simulink model "hex_out"  (Simulink 7.1)
settings: Solver=ode45  StartTime=0.0  StopTime=100000  RelTol=1e-3
InitFcn:
  | init
StartFcn:
  | init
libraries: xbsIndex_r4 x89
settings Model: Creator=sgupta  LastModifiedBy=sgupta

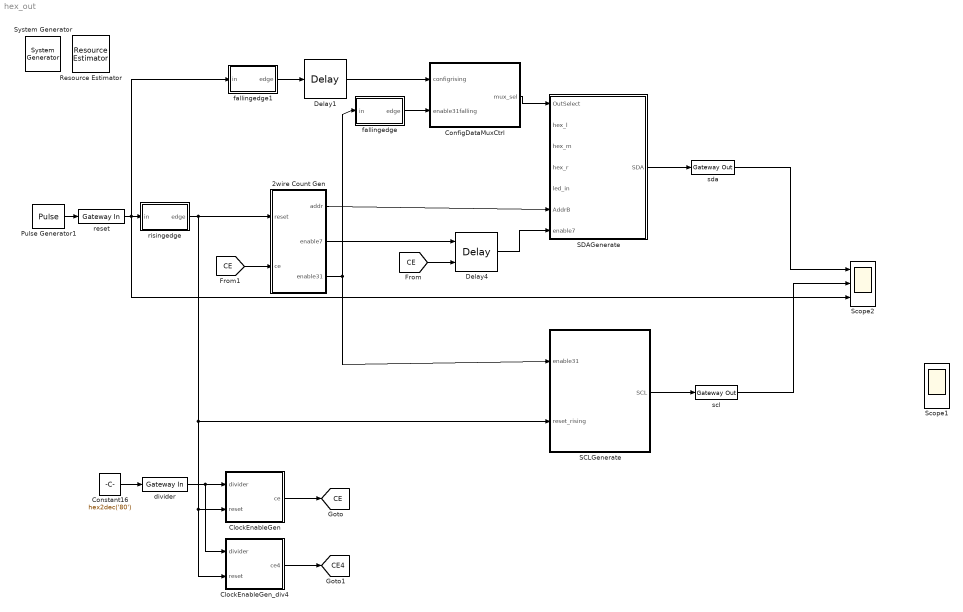
== system hex_out ==
  " System Generator" : xbsIndex_r4/ System Generator  Tag=genX  SystemSampleTime=-1  xilinxfamily=virtex4  part=xc4vfx100  speed=-11  package=ff1517  synthesis_tool=XST  clock_wrapper=Clock Enables  directory=./netlist02  testbench=off  simulink_period=1  sysclk_period=10  dcm_input_clock_period=100  incr_netlist=off  trim_vbits=Everywhere in SubSystem  dbl_ovrd=According to Block Masks  core_generation=According to Block Masks  run_coregen=off  deprecated_control=off  eval_field=0  block_type=sysgen
      settings: block_version=10.1.3
  2wire Count Gen : Subsystem
  ClockEnableGen : Subsystem
  ClockEnableGen_div4 : Subsystem
  ConfigDataMuxCtrl : Subsystem
  Constant16 : Constant  Value=hex2dec('80')  OutDataType=sfix(16)  OutScaling=2^0
  Delay1 : xbsIndex_r4/Delay  en=off  latency=80  dbl_ovrd=off  reg_retiming=off  block_type=delay
      settings: xl_area=[1 1 0 0 0 0 0]
  Delay4 : xbsIndex_r4/Delay  en=on  latency=1  dbl_ovrd=off  reg_retiming=off  block_type=delay
      settings: xl_area=[1 1 0 0 0 0 0]
  Pulse Generator1 : DiscretePulseGenerator  PulseType=Time based  Period=500000  PulseWidth=10/2000*100  PhaseDelay=2000
  Resource Estimator : xbsIndex_r4/Resource Estimator  Tag=resEstTag  Slices=127  FFs=89  BRAMs=0  LUTs=186  IOBs=57  EBMs=0  TBUFs=0  xl_use_estimator_area=off  est_options=Estimate  block_type=resource_estimator
      settings: AttributesFormatString=Resource\nEstimator  block_version=10.1.3
  SCLGenerate : Subsystem
  SDAGenerate : Subsystem
  Scope1 : Scope  NumInputPorts=3
      settings: TimeRange=30000  YMin=0~0~-1  YMax=1~1~1
  Scope2 : Scope  NumInputPorts=3
      settings: YMin=0~0~-1  YMax=1~1~1  SaveName=ScopeData2
  divider : xbsIndex_r4/Gateway In  arith_type=Unsigned  n_bits=8  bin_pt=0  quantization=Truncate  overflow=Wrap  period=1  dbl_ovrd=off  timing_constraint=None  locs_specified=off  LOCs={}  block_type=gatewayin
      settings: infoedit="Gateway in block.  Converts inputs of type Simulink integer, double and fixed point to  Xilinx fixed point type.<P><P>Hardware notes:  In hardware these blocks become top level input ports."  xl_area=[0 0 0 0 8 0 0]  block_version=10.1.3
  fallingedge : Subsystem
  fallingedge1 : Subsystem
  reset : xbsIndex_r4/Gateway In  arith_type=Boolean  n_bits=8  bin_pt=0  quantization=Truncate  overflow=Wrap  period=1  dbl_ovrd=off  timing_constraint=None  locs_specified=off  LOCs={}  block_type=gatewayin
      settings: infoedit="Gateway in block.  Converts inputs of type Simulink integer, double and fixed point to  Xilinx fixed point type.<P><P>Hardware notes:  In hardware these blocks become top level input ports."  xl_area=[0 0 0 0 1 0 0]  block_version=10.1.3
  risingedge : Subsystem
  scl : xbsIndex_r4/Gateway Out  hdl_port=on  timing_constraint=None  locs_specified=off  LOCs={}  block_type=gatewayout
      settings: infoedit="Gateway out block.  Converts Xilinx fixed point inputs into ouputs of type Simulink integer, double, or fixed point.<P><P>Hardware notes:  In hardware these blocks become top level output ports or are discarded, depending on how they are configured."  block_version=10.1.3
  sda : xbsIndex_r4/Gateway Out  hdl_port=on  timing_constraint=None  locs_specified=off  LOCs={}  block_type=gatewayout
      settings: infoedit="Gateway out block.  Converts Xilinx fixed point inputs into ouputs of type Simulink integer, double, or fixed point.<P><P>Hardware notes:  In hardware these blocks become top level output ports or are discarded, depending on how they are configured."  block_version=10.1.3
  tag scope: CE4=global, CE=global
  wires:
  2wire Count Gen/2(enable7) -> Delay4/1
  2wire Count Gen/3(enable31) -> fallingedge/1(in), SCLGenerate/1(enable31)
  divider/1 -> ClockEnableGen/1(divider), ClockEnableGen_div4/1(divider)
  Constant16/1 -> divider/1
  ClockEnableGen/1(ce) -> [CE]
  [CE] -> Delay4/2
  fallingedge/1(edge) -> ConfigDataMuxCtrl/2(enable31falling)
  ClockEnableGen_div4/1(ce4) -> [CE4]
  Delay4/1 -> SDAGenerate/7(enable7)
  2wire Count Gen/1(addr) -> SDAGenerate/6(AddrB)
  ConfigDataMuxCtrl/1(mux_sel) -> SDAGenerate/1(OutSelect)
  [CE] -> 2wire Count Gen/2(ce)
  SDAGenerate/1(SDA) -> sda/1
  SCLGenerate/1(SCL) -> scl/1
  sda/1 -> Scope2/1
  scl/1 -> Scope2/2
  Pulse Generator1/1 -> reset/1
  reset/1 -> Scope2/3, risingedge/1(in), fallingedge1/1(in)
  risingedge/1(edge) -> SCLGenerate/2(reset_rising), ClockEnableGen_div4/2(reset), ClockEnableGen/2(reset), 2wire Count Gen/1(reset)
  fallingedge1/1(edge) -> Delay1/1
  Delay1/1 -> ConfigDataMuxCtrl/1(configrising)

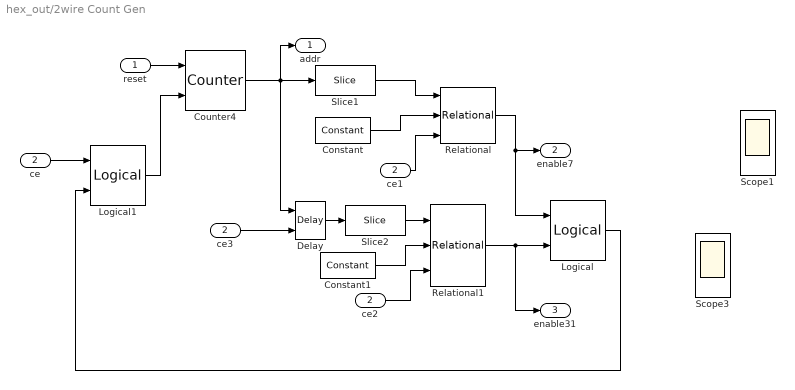
== system hex_out/2wire Count Gen ==
  reset : Inport
  ce : Inport  Port=2
  Constant : xbsIndex_r4/Constant  arith_type=Unsigned  const=7  n_bits=6  bin_pt=0  explicit_period=off  period=1  equ=P=C  opselect=C  inp2=PCIN>>17  opr=+  inp1=P  carry=CIN  dbl_ovrd=off  block_type=constant
  Constant1 : xbsIndex_r4/Constant  arith_type=Unsigned  const=31  n_bits=6  bin_pt=0  explicit_period=off  period=1  equ=P=C  opselect=C  inp2=PCIN>>17  opr=+  inp1=P  carry=CIN  dbl_ovrd=off  block_type=constant
  Counter4 : xbsIndex_r4/Counter  cnt_type=Free Running  cnt_to=23  operation=Up  start_count=0  cnt_by_val=1  arith_type=Unsigned  n_bits=6  bin_pt=0  load_pin=off  rst=on  en=on  explicit_period=on  period=1  dbl_ovrd=off  use_behavioral_HDL=off  use_rpm=off  implementation=Fabric  block_type=counter
      settings: xl_area=[4 6 0 6 0 0 0]
  Delay : xbsIndex_r4/Delay  en=on  latency=1  dbl_ovrd=off  reg_retiming=off  block_type=delay
      settings: xl_area=[3 6 0 0 0 0 0]
  Logical : xbsIndex_r4/Logical  logical_function=AND  inputs=2  en=off  latency=0  precision=Full  arith_type=Unsigned  n_bits=16  bin_pt=0  align_bp=on  dbl_ovrd=off  block_type=logical
      settings: xl_area=[1 0 0 1 0 0 0]
  Logical1 : xbsIndex_r4/Logical  logical_function=AND  inputs=2  en=off  latency=0  precision=Full  arith_type=Unsigned  n_bits=16  bin_pt=0  align_bp=on  dbl_ovrd=off  block_type=logical
      settings: xl_area=[1 0 0 1 0 0 0]
  Relational : xbsIndex_r4/Relational  mode=a!=b  en=on  latency=1  dbl_ovrd=off  block_type=relational
      settings: xl_area=[2 1 0 3 0 0 0]  block_version=10.1.3
  Relational1 : xbsIndex_r4/Relational  mode=a!=b  en=on  latency=1  dbl_ovrd=off  block_type=relational
      settings: xl_area=[2 1 0 3 0 0 0]  block_version=10.1.3
  Scope1 : Scope  NumInputPorts=4
      settings: YMin=-5~-5~-5~-5  YMax=5~5~5~5  SaveName=ScopeData6
  Scope3 : Scope  NumInputPorts=2
      settings: YMin=-5~-5  YMax=5~5  SaveName=ScopeData3
  Slice1 : xbsIndex_r4/Slice  nbits=3  boolean_output=off  mode=Lower Bit Location + Width  bit1=0  base1=MSB of Input  bit0=0  base0=LSB of Input  dbl_ovrd=off  block_type=slice
      settings: infoedit="Extracts a given range of bits from each input sample and presents it at the output.  The output type is ordinarily unsigned with binary point at zero, but can be Boolean when the slice is one bit wide.<P><P>Hardware notes: In hardware this block costs nothing."  block_version=10.1.3
  Slice2 : xbsIndex_r4/Slice  nbits=5  boolean_output=off  mode=Lower Bit Location + Width  bit1=0  base1=MSB of Input  bit0=0  base0=LSB of Input  dbl_ovrd=off  block_type=slice
      settings: infoedit="Extracts a given range of bits from each input sample and presents it at the output.  The output type is ordinarily unsigned with binary point at zero, but can be Boolean when the slice is one bit wide.<P><P>Hardware notes: In hardware this block costs nothing."  block_version=10.1.3
  ce1 : InportShadow  Port=2  LatchByCopyingInsideSignal=off
  ce2 : InportShadow  Port=2  LatchByCopyingInsideSignal=off
  ce3 : InportShadow  Port=2  LatchByCopyingInsideSignal=off
  addr : Outport
  enable7 : Outport  Port=2
  enable31 : Outport  Port=3
  wires:
  Counter4/1 -> addr/1, Delay/1, Slice1/1
  Slice1/1 -> Relational/1
  Constant/1 -> Relational/2
  Relational/1 -> enable7/1, Logical/1
  Constant1/1 -> Relational1/2
  Delay/1 -> Slice2/1
  Relational1/1 -> Logical/2, enable31/1
  Slice2/1 -> Relational1/1
  reset/1 -> Counter4/1
  Logical1/1 -> Counter4/2
  ce/1 -> Logical1/1
  Logical/1 -> Logical1/2
  ce1/1 -> Relational/3
  ce2/1 -> Relational1/3
  ce3/1 -> Delay/2

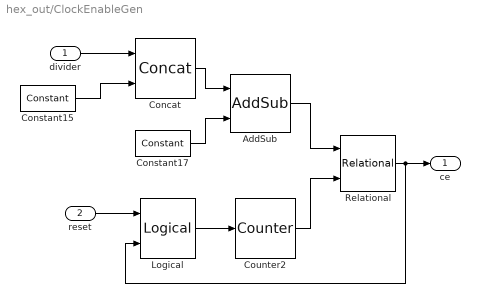
== system hex_out/ClockEnableGen ==
  divider : Inport
  reset : Inport  Port=2
  AddSub : xbsIndex_r4/AddSub  mode=Subtraction  use_carryin=off  use_carryout=off  en=off  latency=0  precision=User Defined  arith_type=Unsigned  n_bits=10  bin_pt=0  quantization=Truncate  overflow=Wrap  dbl_ovrd=off  use_behavioral_HDL=off  pipelined=off  use_rpm=on  hw_selection=Fabric  block_type=addsub
      settings: xl_area=[6 0 0 10 0 0 0]  block_version=10.1.3
  Concat : xbsIndex_r4/Concat  num_inputs=2  dbl_ovrd=off  block_type=concat
      settings: block_version=10.1.3
  Constant15 : xbsIndex_r4/Constant  arith_type=Unsigned  const=0  n_bits=2  bin_pt=0  explicit_period=on  period=1  equ=P=C  opselect=C  inp2=PCIN>>17  opr=+  inp1=P  carry=CIN  dbl_ovrd=off  block_type=constant
  Constant17 : xbsIndex_r4/Constant  arith_type=Unsigned  const=2  n_bits=10  bin_pt=0  explicit_period=on  period=1  equ=P=C  opselect=C  inp2=PCIN>>17  opr=+  inp1=P  carry=CIN  dbl_ovrd=off  block_type=constant
  Counter2 : xbsIndex_r4/Counter  cnt_type=Free Running  cnt_to=23  operation=Up  start_count=0  cnt_by_val=1  arith_type=Unsigned  n_bits=10  bin_pt=0  load_pin=off  rst=on  en=off  explicit_period=on  period=1  dbl_ovrd=off  use_behavioral_HDL=off  use_rpm=off  implementation=Fabric  block_type=counter
      settings: xl_area=[6 10 0 10 0 0 0]
  Logical : xbsIndex_r4/Logical  logical_function=OR  inputs=2  en=off  latency=0  precision=Full  arith_type=Unsigned  n_bits=16  bin_pt=0  align_bp=on  dbl_ovrd=off  block_type=logical
  Relational : xbsIndex_r4/Relational  mode=a=b  en=off  latency=1  dbl_ovrd=off  block_type=relational
      settings: xl_area=[3 1 0 6 0 0 0]  block_version=10.1.3
  ce : Outport
  wires:
  Constant15/1 -> Concat/2
  Counter2/1 -> Relational/2
  Relational/1 -> ce/1, Logical/2
  AddSub/1 -> Relational/1
  Concat/1 -> AddSub/1
  Constant17/1 -> AddSub/2
  divider/1 -> Concat/1
  Logical/1 -> Counter2/1
  reset/1 -> Logical/1

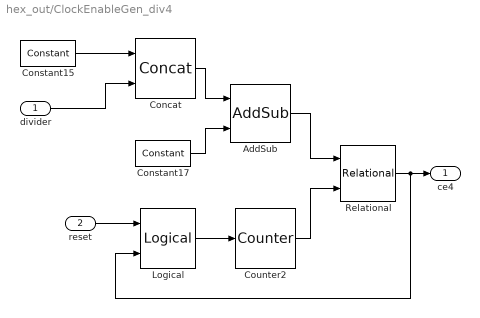
== system hex_out/ClockEnableGen_div4 ==
  divider : Inport
  reset : Inport  Port=2
  AddSub : xbsIndex_r4/AddSub  mode=Subtraction  use_carryin=off  use_carryout=off  en=off  latency=0  precision=User Defined  arith_type=Unsigned  n_bits=10  bin_pt=0  quantization=Truncate  overflow=Wrap  dbl_ovrd=off  use_behavioral_HDL=off  pipelined=off  use_rpm=on  hw_selection=Fabric  block_type=addsub
      settings: xl_area=[6 0 0 10 0 0 0]  block_version=10.1.3
  Concat : xbsIndex_r4/Concat  num_inputs=2  dbl_ovrd=off  block_type=concat
      settings: block_version=10.1.3
  Constant15 : xbsIndex_r4/Constant  arith_type=Unsigned  const=0  n_bits=2  bin_pt=0  explicit_period=on  period=1  equ=P=C  opselect=C  inp2=PCIN>>17  opr=+  inp1=P  carry=CIN  dbl_ovrd=off  block_type=constant
  Constant17 : xbsIndex_r4/Constant  arith_type=Unsigned  const=2  n_bits=10  bin_pt=0  explicit_period=on  period=1  equ=P=C  opselect=C  inp2=PCIN>>17  opr=+  inp1=P  carry=CIN  dbl_ovrd=off  block_type=constant
  Counter2 : xbsIndex_r4/Counter  cnt_type=Free Running  cnt_to=23  operation=Up  start_count=0  cnt_by_val=1  arith_type=Unsigned  n_bits=10  bin_pt=0  load_pin=off  rst=on  en=off  explicit_period=on  period=1  dbl_ovrd=off  use_behavioral_HDL=off  use_rpm=off  implementation=Fabric  block_type=counter
      settings: xl_area=[6 10 0 10 0 0 0]
  Logical : xbsIndex_r4/Logical  logical_function=OR  inputs=2  en=off  latency=0  precision=Full  arith_type=Unsigned  n_bits=16  bin_pt=0  align_bp=on  dbl_ovrd=off  block_type=logical
  Relational : xbsIndex_r4/Relational  mode=a=b  en=off  latency=1  dbl_ovrd=off  block_type=relational
      settings: xl_area=[3 1 0 6 0 0 0]  block_version=10.1.3
  ce4 : Outport
  wires:
  Constant17/1 -> AddSub/2
  AddSub/1 -> Relational/1
  Relational/1 -> ce4/1, Logical/2
  Counter2/1 -> Relational/2
  Concat/1 -> AddSub/1
  Constant15/1 -> Concat/1
  divider/1 -> Concat/2
  Logical/1 -> Counter2/1
  reset/1 -> Logical/1

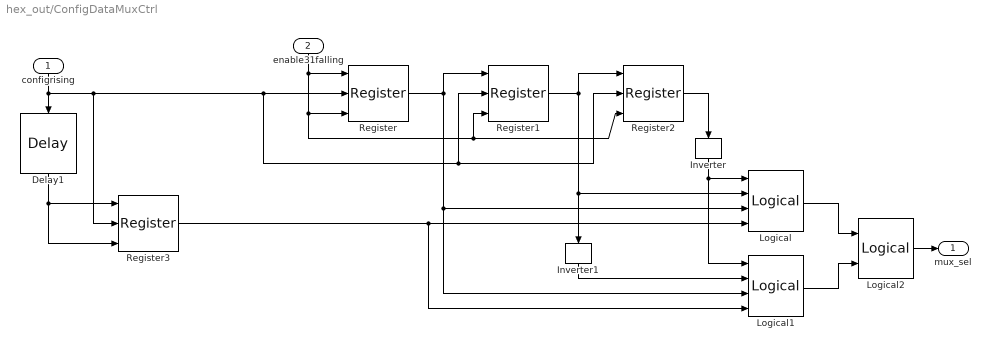
== system hex_out/ConfigDataMuxCtrl ==
  configrising : Inport  Orientation=down
  enable31falling : Inport  Orientation=down  Port=2
  Delay1 : xbsIndex_r4/Delay  Orientation=down  en=off  latency=1  dbl_ovrd=off  reg_retiming=off  block_type=delay
      settings: xl_area=[1 1 0 0 0 0 0]
  Inverter : xbsIndex_r4/Inverter  Orientation=down  en=off  latency=0  dbl_ovrd=off  block_type=inv
      settings: xl_area=[0 0 0 0 0 0 0]
  Inverter1 : xbsIndex_r4/Inverter  Orientation=down  en=off  latency=0  dbl_ovrd=off  block_type=inv
      settings: xl_area=[0 0 0 0 0 0 0]
  Logical : xbsIndex_r4/Logical  logical_function=AND  inputs=4  en=off  latency=0  precision=Full  arith_type=Unsigned  n_bits=16  bin_pt=0  align_bp=on  dbl_ovrd=off  block_type=logical
      settings: xl_area=[1 0 0 1 0 0 0]
  Logical1 : xbsIndex_r4/Logical  logical_function=AND  inputs=4  en=off  latency=0  precision=Full  arith_type=Unsigned  n_bits=16  bin_pt=0  align_bp=on  dbl_ovrd=off  block_type=logical
      settings: xl_area=[1 0 0 1 0 0 0]
  Logical2 : xbsIndex_r4/Logical  logical_function=OR  inputs=2  en=off  latency=0  precision=Full  arith_type=Unsigned  n_bits=16  bin_pt=0  align_bp=on  dbl_ovrd=off  block_type=logical
      settings: xl_area=[1 0 0 1 0 0 0]
  Register{,1..3} (4 alike) : xbsIndex_r4/Register  init=0  rst=on  en=on  dbl_ovrd=off  block_type=register
      settings: xl_area=[1 1 0 0 0 0 0]
  mux_sel : Outport
  wires:
  enable31falling/1 -> Register2/3, Register1/3, Register/3, Register/1
  Register/1 -> Register1/1, Logical/3, Logical1/3
  Register1/1 -> Register2/1, Logical/2, Inverter1/1
  Delay1/1 -> Register3/1, Register3/3
  Register2/1 -> Inverter/1
  Register3/1 -> Logical/4, Logical1/4
  Inverter/1 -> Logical/1, Logical1/1
  Inverter1/1 -> Logical1/2
  Logical/1 -> Logical2/1
  Logical1/1 -> Logical2/2
  configrising/1 -> Delay1/1, Register/2, Register1/2, Register2/2, Register3/2
  Logical2/1 -> mux_sel/1

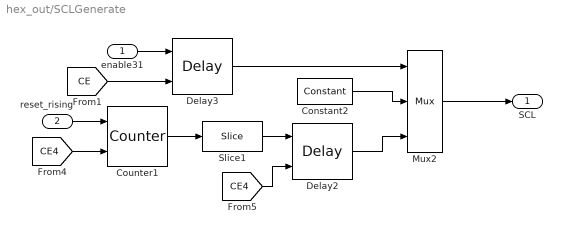
== system hex_out/SCLGenerate ==
  enable31 : Inport
  reset_rising : Inport  Port=2
  Constant2 : xbsIndex_r4/Constant  arith_type=Unsigned  const=1  n_bits=1  bin_pt=0  explicit_period=off  period=1  equ=P=C  opselect=C  inp2=PCIN>>17  opr=+  inp1=P  carry=CIN  dbl_ovrd=off  block_type=constant
  Counter1 : xbsIndex_r4/Counter  cnt_type=Free Running  cnt_to=23  operation=Up  start_count=0  cnt_by_val=1  arith_type=Unsigned  n_bits=2  bin_pt=0  load_pin=off  rst=on  en=on  explicit_period=on  period=1  dbl_ovrd=off  use_behavioral_HDL=off  use_rpm=off  implementation=Fabric  block_type=counter
      settings: xl_area=[2 2 0 2 0 0 0]
  Delay2 : xbsIndex_r4/Delay  en=on  latency=4  dbl_ovrd=off  reg_retiming=off  block_type=delay
      settings: xl_area=[1 1 0 1 0 0 0]
  Delay3 : xbsIndex_r4/Delay  en=on  latency=1  dbl_ovrd=off  reg_retiming=off  block_type=delay
      settings: xl_area=[1 1 0 0 0 0 0]
  Mux2 : xbsIndex_r4/Mux  inputs=2  en=off  latency=0  precision=Full  arith_type=Unsigned  n_bits=16  bin_pt=14  quantization=Truncate  overflow=Wrap  dbl_ovrd=off  block_type=mux
      settings: xl_area=[1 0 0 1 0 0 0]
  Slice1 : xbsIndex_r4/Slice  nbits=1  boolean_output=off  mode=Upper Bit Location + Width  bit1=0  base1=MSB of Input  bit0=0  base0=LSB of Input  dbl_ovrd=off  block_type=slice
      settings: infoedit="Extracts a given range of bits from each input sample and presents it at the output.  The output type is ordinarily unsigned with binary point at zero, but can be Boolean when the slice is one bit wide.<P><P>Hardware notes: In hardware this block costs nothing."  block_version=10.1.3
  SCL : Outport
  wires:
  Counter1/1 -> Slice1/1
  Slice1/1 -> Delay2/1
  Delay2/1 -> Mux2/3
  Constant2/1 -> Mux2/2
  [CE] -> Delay3/2
  Delay3/1 -> Mux2/1
  [CE4] -> Counter1/2
  [CE4] -> Delay2/2
  enable31/1 -> Delay3/1
  reset_rising/1 -> Counter1/1
  Mux2/1 -> SCL/1

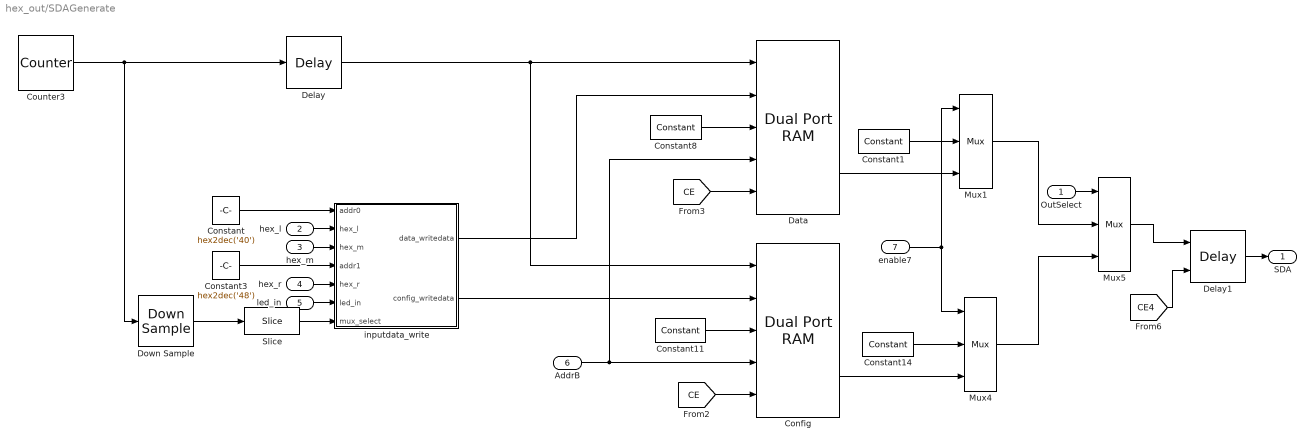
== system hex_out/SDAGenerate ==
  OutSelect : Inport
  hex_l : Inport  Port=2
  hex_m : Inport  Port=3
  hex_r : Inport  Port=4
  led_in : Inport  Port=5
  AddrB : Inport  Port=6
  enable7 : Inport  Port=7
  Config : xbsIndex_r4/Dual Port RAM  depth=64  initVector=0  distributed_mem=Distributed memory  init_a=0  init_b=0  rst_a=off  rst_b=off  en_a=off  en_b=on  latency=1  write_mode_A=Read After Write  write_mode_B=Read Before Write  dbl_ovrd=off  optimize=Area  use_rpm=on  block_type=dpram
      settings: xl_area=[4 2 0 8 0 0 0]  block_version=10.1.3
  Constant : Constant  Value=hex2dec('40')  OutDataType=sfix(16)  OutScaling=2^0
  Constant1 : xbsIndex_r4/Constant  arith_type=Unsigned  const=1  n_bits=1  bin_pt=0  explicit_period=off  period=1  equ=P=C  opselect=C  inp2=PCIN>>17  opr=+  inp1=P  carry=CIN  dbl_ovrd=off  block_type=constant
  Constant11 : xbsIndex_r4/Constant  arith_type=Boolean  const=1  n_bits=1  bin_pt=0  explicit_period=off  period=1  equ=P=C  opselect=C  inp2=PCIN>>17  opr=+  inp1=P  carry=CIN  dbl_ovrd=off  block_type=constant
  Constant14 : xbsIndex_r4/Constant  arith_type=Unsigned  const=1  n_bits=1  bin_pt=0  explicit_period=off  period=1  equ=P=C  opselect=C  inp2=PCIN>>17  opr=+  inp1=P  carry=CIN  dbl_ovrd=off  block_type=constant
  Constant3 : Constant  Value=hex2dec('48')  OutDataType=sfix(16)  OutScaling=2^0
  Constant8 : xbsIndex_r4/Constant  arith_type=Boolean  const=1  n_bits=1  bin_pt=0  explicit_period=off  period=1  equ=P=C  opselect=C  inp2=PCIN>>17  opr=+  inp1=P  carry=CIN  dbl_ovrd=off  block_type=constant
  Counter3 : xbsIndex_r4/Counter  cnt_type=Free Running  cnt_to=23  operation=Up  start_count=0  cnt_by_val=1  arith_type=Unsigned  n_bits=6  bin_pt=0  load_pin=off  rst=off  en=off  explicit_period=on  period=1  dbl_ovrd=off  use_behavioral_HDL=off  use_rpm=off  implementation=Fabric  block_type=counter
      settings: xl_area=[4 6 0 6 0 0 0]
  Data : xbsIndex_r4/Dual Port RAM  depth=64  initVector=0  distributed_mem=Distributed memory  init_a=0  init_b=0  rst_a=off  rst_b=off  en_a=off  en_b=on  latency=1  write_mode_A=Read After Write  write_mode_B=Read Before Write  dbl_ovrd=off  optimize=Area  use_rpm=on  block_type=dpram
      settings: xl_area=[4 2 0 8 0 0 0]  block_version=10.1.3
  Delay : xbsIndex_r4/Delay  en=off  latency=8  dbl_ovrd=off  reg_retiming=off  block_type=delay
      settings: xl_area=[3 6 0 6 0 0 0]
  Delay1 : xbsIndex_r4/Delay  en=on  latency=1  dbl_ovrd=off  reg_retiming=off  block_type=delay
      settings: xl_area=[1 1 0 0 0 0 0]
  Down Sample : xbsIndex_r4/Down Sample  sample_ratio=8  sample_phase="Last Value of Frame  (most efficient)"  en=off  latency=1  dbl_ovrd=off  block_type=dsamp
      settings: xl_area=[3 6 0 0 0 0 0]  block_version=10.1.3
  Mux1 : xbsIndex_r4/Mux  inputs=2  en=off  latency=0  precision=Full  arith_type=Unsigned  n_bits=16  bin_pt=14  quantization=Truncate  overflow=Wrap  dbl_ovrd=off  block_type=mux
      settings: xl_area=[1 0 0 1 0 0 0]
  Mux4 : xbsIndex_r4/Mux  inputs=2  en=off  latency=0  precision=Full  arith_type=Unsigned  n_bits=16  bin_pt=14  quantization=Truncate  overflow=Wrap  dbl_ovrd=off  block_type=mux
      settings: xl_area=[1 0 0 1 0 0 0]
  Mux5 : xbsIndex_r4/Mux  inputs=2  en=off  latency=0  precision=Full  arith_type=Unsigned  n_bits=16  bin_pt=14  quantization=Truncate  overflow=Wrap  dbl_ovrd=off  block_type=mux
      settings: xl_area=[1 0 0 1 0 0 0]
  Slice : xbsIndex_r4/Slice  nbits=3  boolean_output=off  mode=Upper Bit Location + Width  bit1=0  base1=MSB of Input  bit0=0  base0=LSB of Input  dbl_ovrd=off  block_type=slice
      settings: infoedit="Extracts a given range of bits from each input sample and presents it at the output.  The output type is ordinarily unsigned with binary point at zero, but can be Boolean when the slice is one bit wide.<P><P>Hardware notes: In hardware this block costs nothing."  block_version=10.1.3
  inputdata_write : Subsystem
  SDA : Outport
  wires:
  Counter3/1 -> Down Sample/1, Delay/1
  Constant8/1 -> Data/3
  inputdata_write/1(data_writedata) -> Data/2
  Down Sample/1 -> Slice/1
  AddrB/1 -> Data/4, Config/4
  Data/2 -> Mux1/3
  Constant1/1 -> Mux1/2
  Constant/1 -> inputdata_write/1(addr0)
  Constant3/1 -> inputdata_write/4(addr1)
  inputdata_write/2(config_writedata) -> Config/2
  Constant11/1 -> Config/3
  Config/2 -> Mux4/3
  Constant14/1 -> Mux4/2
  Mux1/1 -> Mux5/2
  Mux4/1 -> Mux5/3
  Delay/1 -> Data/1, Config/1
  Slice/1 -> inputdata_write/7(mux_select)
  [CE] -> Config/5
  [CE] -> Data/5
  Mux5/1 -> Delay1/1
  [CE4] -> Delay1/2
  OutSelect/1 -> Mux5/1
  hex_l/1 -> inputdata_write/2(hex_l)
  hex_m/1 -> inputdata_write/3(hex_m)
  Delay1/1 -> SDA/1
  hex_r/1 -> inputdata_write/5(hex_r)
  led_in/1 -> inputdata_write/6(led_in)
  enable7/1 -> Mux1/1, Mux4/1

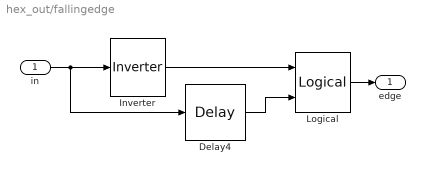
== system hex_out/fallingedge ==
  in : Inport
  Delay4 : xbsIndex_r4/Delay  en=off  latency=1  dbl_ovrd=off  reg_retiming=off  block_type=delay
      settings: xl_area=[1 1 0 0 0 0 0]
  Inverter : xbsIndex_r4/Inverter  en=off  latency=0  dbl_ovrd=off  block_type=inv
      settings: xl_area=[0 0 0 0 0 0 0]
  Logical : xbsIndex_r4/Logical  logical_function=AND  inputs=2  en=off  latency=0  precision=Full  arith_type=Unsigned  n_bits=16  bin_pt=0  align_bp=on  dbl_ovrd=off  block_type=logical
      settings: xl_area=[1 0 0 1 0 0 0]
  edge : Outport
  wires:
  Logical/1 -> edge/1
  Delay4/1 -> Logical/2
  in/1 -> Inverter/1, Delay4/1
  Inverter/1 -> Logical/1

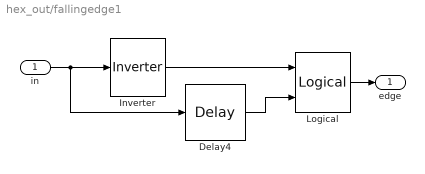
== system hex_out/fallingedge1 ==
  in : Inport
  Delay4 : xbsIndex_r4/Delay  en=off  latency=1  dbl_ovrd=off  reg_retiming=off  block_type=delay
      settings: xl_area=[1 1 0 0 0 0 0]
  Inverter : xbsIndex_r4/Inverter  en=off  latency=0  dbl_ovrd=off  block_type=inv
      settings: xl_area=[0 0 0 0 0 0 0]
  Logical : xbsIndex_r4/Logical  logical_function=AND  inputs=2  en=off  latency=0  precision=Full  arith_type=Unsigned  n_bits=16  bin_pt=0  align_bp=on  dbl_ovrd=off  block_type=logical
      settings: xl_area=[1 0 0 1 0 0 0]
  edge : Outport
  wires:
  Inverter/1 -> Logical/1
  in/1 -> Delay4/1, Inverter/1
  Delay4/1 -> Logical/2
  Logical/1 -> edge/1

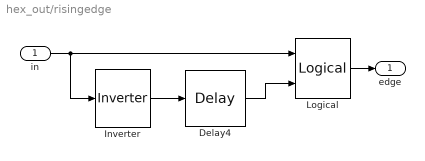
== system hex_out/risingedge ==
  in : Inport
  Delay4 : xbsIndex_r4/Delay  en=off  latency=1  dbl_ovrd=off  reg_retiming=off  block_type=delay
      settings: xl_area=[1 1 0 0 0 0 0]
  Inverter : xbsIndex_r4/Inverter  en=off  latency=0  dbl_ovrd=off  block_type=inv
      settings: xl_area=[0 0 0 0 0 0 0]
  Logical : xbsIndex_r4/Logical  logical_function=AND  inputs=2  en=off  latency=0  precision=Full  arith_type=Unsigned  n_bits=16  bin_pt=0  align_bp=on  dbl_ovrd=off  block_type=logical
      settings: xl_area=[1 0 0 1 0 0 0]
  edge : Outport
  wires:
  in/1 -> Logical/1, Inverter/1
  Inverter/1 -> Delay4/1
  Delay4/1 -> Logical/2
  Logical/1 -> edge/1

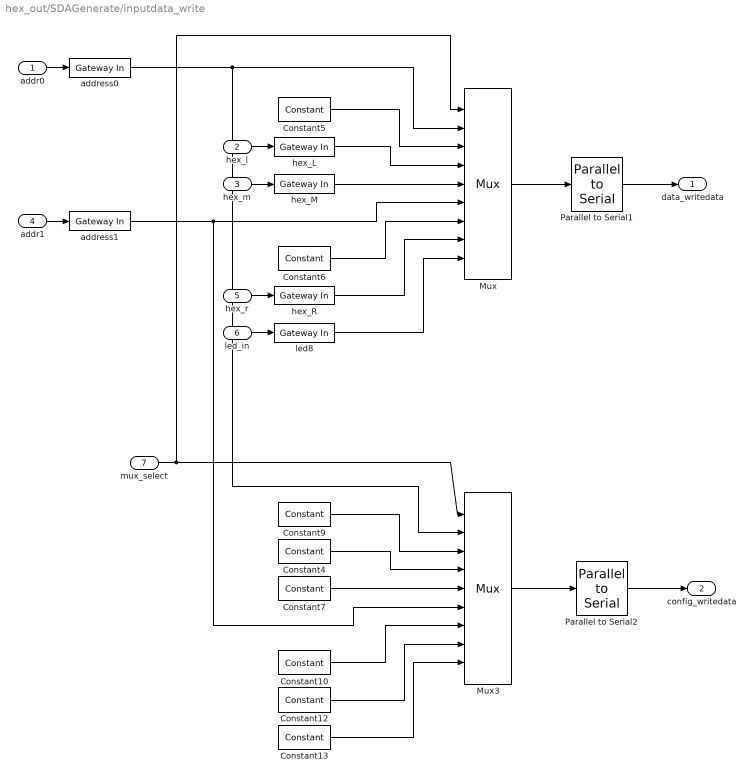
== system hex_out/SDAGenerate/inputdata_write ==
  addr0 : Inport
  hex_l : Inport  Port=2
  hex_m : Inport  Port=3
  addr1 : Inport  Port=4
  hex_r : Inport  Port=5
  led_in : Inport  Port=6
  mux_select : Inport  Port=7
  Constant10 : xbsIndex_r4/Constant  arith_type=Unsigned  const=6  n_bits=8  bin_pt=0  explicit_period=on  period=8  equ=P=C  opselect=C  inp2=PCIN>>17  opr=+  inp1=P  carry=CIN  dbl_ovrd=off  block_type=constant
  Constant{4,7,12..13} (4 alike) : xbsIndex_r4/Constant  arith_type=Unsigned  const=0  n_bits=8  bin_pt=0  explicit_period=on  period=8  equ=P=C  opselect=C  inp2=PCIN>>17  opr=+  inp1=P  carry=CIN  dbl_ovrd=off  block_type=constant
  Constant5 : xbsIndex_r4/Constant  arith_type=Unsigned  const=2  n_bits=8  bin_pt=0  explicit_period=on  period=8  equ=P=C  opselect=C  inp2=PCIN>>17  opr=+  inp1=P  carry=CIN  dbl_ovrd=off  block_type=constant
  Constant6 : xbsIndex_r4/Constant  arith_type=Unsigned  const=2  n_bits=8  bin_pt=0  explicit_period=on  period=8  equ=P=C  opselect=C  inp2=PCIN>>17  opr=+  inp1=P  carry=CIN  dbl_ovrd=off  block_type=constant
  Constant9 : xbsIndex_r4/Constant  arith_type=Unsigned  const=6  n_bits=8  bin_pt=0  explicit_period=on  period=8  equ=P=C  opselect=C  inp2=PCIN>>17  opr=+  inp1=P  carry=CIN  dbl_ovrd=off  block_type=constant
  Mux : xbsIndex_r4/Mux  inputs=8  en=off  latency=0  precision=Full  arith_type=Unsigned  n_bits=16  bin_pt=14  quantization=Truncate  overflow=Wrap  dbl_ovrd=off  block_type=mux
      settings: xl_area=[16 0 0 32 0 0 0]
  Mux3 : xbsIndex_r4/Mux  inputs=8  en=off  latency=0  precision=Full  arith_type=Unsigned  n_bits=16  bin_pt=14  quantization=Truncate  overflow=Wrap  dbl_ovrd=off  block_type=mux
      settings: xl_area=[16 0 0 32 0 0 0]
  Parallel to Serial1 : xbsIndex_r4/Parallel to Serial  output_order=Most Significant Word First  arith_type=Unsigned  output_bits=1  bin_pt=0  en=off  latency=0  dbl_ovrd=off  block_type=p2s
      settings: infoedit=Each sample presented at the input becomes several samples presented serially at the output.  xl_area=[6 9 0 8 0 0 0]  block_version=10.1.3
  Parallel to Serial2 : xbsIndex_r4/Parallel to Serial  output_order=Most Significant Word First  arith_type=Unsigned  output_bits=1  bin_pt=0  en=off  latency=0  dbl_ovrd=off  block_type=p2s
      settings: infoedit=Each sample presented at the input becomes several samples presented serially at the output.  xl_area=[6 9 0 8 0 0 0]  block_version=10.1.3
  address0 : xbsIndex_r4/Gateway In  arith_type=Unsigned  n_bits=8  bin_pt=0  quantization=Truncate  overflow=Wrap  period=8  dbl_ovrd=off  timing_constraint=None  locs_specified=off  LOCs={}  block_type=gatewayin
      settings: infoedit="Gateway in block.  Converts inputs of type Simulink integer, double and fixed point to  Xilinx fixed point type.<P><P>Hardware notes:  In hardware these blocks become top level input ports."  xl_area=[0 0 0 0 8 0 0]  block_version=10.1.3
  address1 : xbsIndex_r4/Gateway In  arith_type=Unsigned  n_bits=8  bin_pt=0  quantization=Truncate  overflow=Wrap  period=8  dbl_ovrd=off  timing_constraint=None  locs_specified=off  LOCs={}  block_type=gatewayin
      settings: infoedit="Gateway in block.  Converts inputs of type Simulink integer, double and fixed point to  Xilinx fixed point type.<P><P>Hardware notes:  In hardware these blocks become top level input ports."  xl_area=[0 0 0 0 8 0 0]  block_version=10.1.3
  hex_L : xbsIndex_r4/Gateway In  arith_type=Unsigned  n_bits=8  bin_pt=0  quantization=Truncate  overflow=Wrap  period=8  dbl_ovrd=off  timing_constraint=None  locs_specified=off  LOCs={}  block_type=gatewayin
      settings: infoedit="Gateway in block.  Converts inputs of type Simulink integer, double and fixed point to  Xilinx fixed point type.<P><P>Hardware notes:  In hardware these blocks become top level input ports."  xl_area=[0 0 0 0 8 0 0]  block_version=10.1.3
  hex_M : xbsIndex_r4/Gateway In  arith_type=Unsigned  n_bits=8  bin_pt=0  quantization=Truncate  overflow=Wrap  period=8  dbl_ovrd=off  timing_constraint=None  locs_specified=off  LOCs={}  block_type=gatewayin
      settings: infoedit="Gateway in block.  Converts inputs of type Simulink integer, double and fixed point to  Xilinx fixed point type.<P><P>Hardware notes:  In hardware these blocks become top level input ports."  xl_area=[0 0 0 0 8 0 0]  block_version=10.1.3
  hex_R : xbsIndex_r4/Gateway In  arith_type=Unsigned  n_bits=8  bin_pt=0  quantization=Truncate  overflow=Wrap  period=8  dbl_ovrd=off  timing_constraint=None  locs_specified=off  LOCs={}  block_type=gatewayin
      settings: infoedit="Gateway in block.  Converts inputs of type Simulink integer, double and fixed point to  Xilinx fixed point type.<P><P>Hardware notes:  In hardware these blocks become top level input ports."  xl_area=[0 0 0 0 8 0 0]  block_version=10.1.3
  led8 : xbsIndex_r4/Gateway In  arith_type=Unsigned  n_bits=8  bin_pt=0  quantization=Truncate  overflow=Wrap  period=8  dbl_ovrd=off  timing_constraint=None  locs_specified=off  LOCs={}  block_type=gatewayin
      settings: infoedit="Gateway in block.  Converts inputs of type Simulink integer, double and fixed point to  Xilinx fixed point type.<P><P>Hardware notes:  In hardware these blocks become top level input ports."  xl_area=[0 0 0 0 8 0 0]  block_version=10.1.3
  data_writedata : Outport
  config_writedata : Outport  Port=2
  wires:
  address0/1 -> Mux/2, Mux3/2
  Constant5/1 -> Mux/3
  hex_L/1 -> Mux/4
  hex_M/1 -> Mux/5
  address1/1 -> Mux/6, Mux3/6
  Constant6/1 -> Mux/7
  hex_R/1 -> Mux/8
  led8/1 -> Mux/9
  Mux/1 -> Parallel to Serial1/1
  Constant9/1 -> Mux3/3
  Constant4/1 -> Mux3/4
  Constant7/1 -> Mux3/5
  Constant10/1 -> Mux3/7
  Constant12/1 -> Mux3/8
  Constant13/1 -> Mux3/9
  Mux3/1 -> Parallel to Serial2/1
  mux_select/1 -> Mux3/1, Mux/1
  addr0/1 -> address0/1
  hex_l/1 -> hex_L/1
  Parallel to Serial1/1 -> data_writedata/1
  hex_m/1 -> hex_M/1
  addr1/1 -> address1/1
  hex_r/1 -> hex_R/1
  led_in/1 -> led8/1
  Parallel to Serial2/1 -> config_writedata/1
